simulink model "pid_demo"  (R2025b)
settings: Solver=VariableStepAuto  StartTime=0.0  StopTime=50  RelTol=1e-3
PostLoadFcn:
  | pid_demo_init
values from neighbouring files (symbols this model uses):
  A = [0, 0, 1, 0 ... (first row only)    [IP2_init.m]    (also in IP3_init.m; IP4_init.m; IP_init.m; pid_demo_init.m = [0, 0, 0)
  B = [0;0;4/ (4 * M + m); 6 / (l * (4 * M + m))]    [IP2_init.m]    (also in IP3_init.m; IP4_init.m; IP_init.m; pid_demo_init.m = [1; kd / (Tf + Ts); ki * Ts])
  C = [1, 0, 0, 0]    [IP2_init.m]    (also in IP3_init.m; IP4_init.m; IP_init.m; pid_demo_init.m = [-kd / (Tf + Ts), Tf / (Tf + Ts), 1])
  D = 0    [IP2_init.m]    (also in IP3_init.m; IP4_init.m; IP_init.m; pid_demo_init.m = 333.833333333)
  Ts = 1e-2    (= 0.01)    [IP4_init.m]    (also in pid_demo_init.m; rcm_generator.m = block.DialogPrm(2).Data)
settings Model: Creator=Junch  LastModifiedBy=Junch

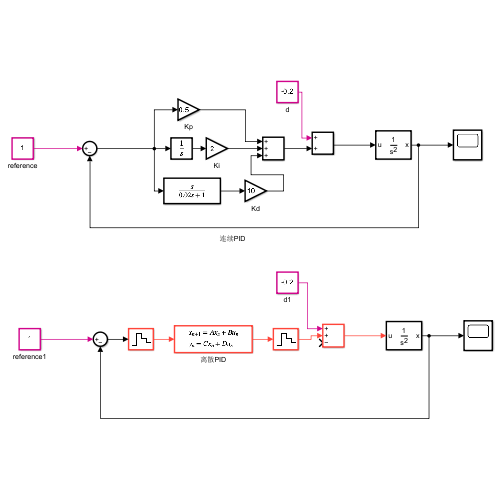
[thumbnail: Simulink's stored preview of the top-level diagram]
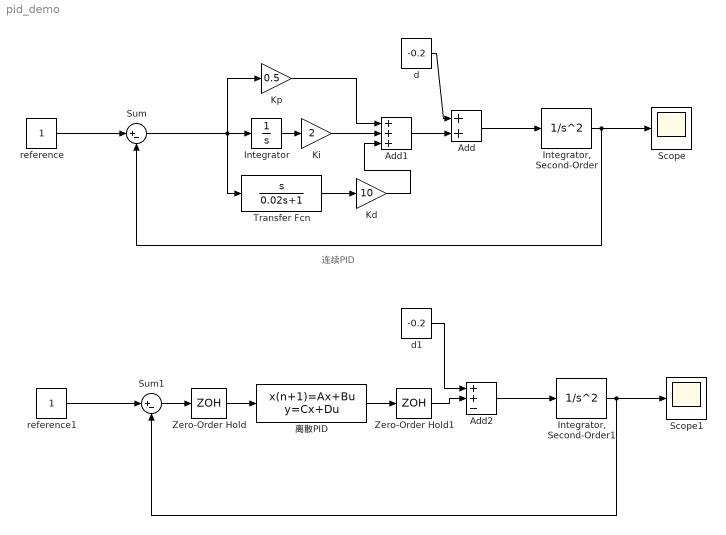
== system pid_demo ==
  note: 连续PID
  Add : Sum
  Add1 : Sum  Inputs=+++
  Add2 : Sum  Inputs=++-
  Integrator : Integrator
  "Integrator, Second-Order" : SecondOrderIntegrator  ShowOutput=x
  "Integrator, Second-Order1" : SecondOrderIntegrator  ShowOutput=x
  Kd : Gain  Gain=10
  Ki : Gain  Gain=2
  Kp : Gain  Gain=0.5
  Scope : Scope
      settings: ActiveDisplayYMinimum=-1  ActiveDisplayYMaximum=1
  Scope1 : Scope
      settings: ActiveDisplayYMinimum=-0.12543685088308018  ActiveDisplayYMaximum=1.1289316579477218
  Sum : Sum  Inputs=|+-
  Sum1 : Sum  Inputs=|+-
  Transfer Fcn : TransferFcn  Numerator=[1 0]  Denominator=[0.02 1]
  Zero-Order Hold : ZeroOrderHold  SampleTime=Ts
  Zero-Order Hold1 : ZeroOrderHold  SampleTime=Ts
  d : Constant  Value=-0.2
  d1 : Constant  Value=-0.2
  reference : Constant
  reference1 : Constant
  离散PID : DiscreteStateSpace  A=A  B=B  C=C  D=D  SampleTime=Ts
  wires:
  Kp/1 -> Add1/1
  "Integrator, Second-Order"/1 -> Sum/2, Scope/1
  Sum/1 -> Kp/1, Transfer Fcn/1, Integrator/1
  reference/1 -> Sum/1
  Add/1 -> "Integrator, Second-Order"/1
  d/1 -> Add/1
  Add1/1 -> Add/2
  Transfer Fcn/1 -> Kd/1
  Kd/1 -> Add1/3
  Integrator/1 -> Ki/1
  Ki/1 -> Add1/2
  "Integrator, Second-Order1"/1 -> Sum1/2, Scope1/1
  d1/1 -> Add2/1
  Add2/1 -> "Integrator, Second-Order1"/1
  Sum1/1 -> Zero-Order Hold/1
  离散PID/1 -> Zero-Order Hold1/1
  Zero-Order Hold/1 -> 离散PID/1
  Zero-Order Hold1/1 -> Add2/2
  reference1/1 -> Sum1/1
